simulink model "gm_Encoder_Zynq_vnl"  (R2018a)
settings: Solver=ode3  StartTime=0.0  StopTime=SimulationsDauer  RelTol=1e-3  EnableMultiTasking=on
undefined symbols (not defined in the file or in its folder): DiscIntNeverNeededParam, f_ISR, IncPerTurn, n_max, OverSamplingFactor, OverSamplingFactorInverse, Periode, Phase_Delay_A, Phase_Delay_B, PolePair, T_mech, TestDrehzahl_rpm
libraries: simulink x18, hdlsllib x2, dspsigops x2, dspswit3 x2, powerlib_meascontrol x2, hdlmdlgenlib x1, simulink_extras x1, powerlib x1
(part 3 of 3)

== system gm_Encoder_Zynq_vnl/IncreEncoder_V22/Check_Direction ==
  A : Inport  PortDimensions=1  SampleTime=2e-08
  B : Inport  Port=2  PortDimensions=1  SampleTime=2e-08
  Add : Sum  Inputs=+-  AccumDataTypeStr=fixdt(1, 4, 0)  OutDataTypeStr=fixdt(1, 4, 0)  SampleTime=2e-08
  Add1 : Sum  Inputs=+-  AccumDataTypeStr=fixdt(1, 4, 0)  OutDataTypeStr=fixdt(1, 4, 0)  SampleTime=2e-08
  Add2 : Sum  AccumDataTypeStr=fixdt(1, 4, 0)  OutDataTypeStr=fixdt(1, 4, 0)  SampleTime=2e-08
  Change : Sum  AccumDataTypeStr=fixdt(1, 4, 0)  OutDataTypeStr=fixdt(1, 4, 0)  SampleTime=2e-08
  Change1 : Delay  DelayLength=double(1)  InitialCondition=0  InputProcessing=Inherited  SampleTime=2e-08
  Save_Direction : Switch  Criteria=u2 ~= 0  Threshold=double(0)  OutDataTypeStr=fixdt(1, 4, 0)  SampleTime=2e-08
  T_count_switch : Switch  Threshold=double(1)  OutDataTypeStr=fixdt(1, 4, 0)  SampleTime=2e-08
  TrnLeft : Sum  Inputs=+-  AccumDataTypeStr=fixdt(1, 4, 0)  OutDataTypeStr=fixdt(1, 4, 0)  SampleTime=2e-08
  TrnRight : Sum  Inputs=+-  AccumDataTypeStr=fixdt(1, 4, 0)  OutDataTypeStr=fixdt(1, 4, 0)  SampleTime=2e-08
  TurnLeft : Constant  Value=fi(0,1,4,0,'hex','f')  OutDataTypeStr=fixdt(1, 4, 0)  SampleTime=-1
  TurnRight : Constant  Value=fi(0,1,4,0,'hex','1')  OutDataTypeStr=fixdt(1, 4, 0)  SampleTime=-1
  count_old : Delay  DelayLength=double(1)  InitialCondition=0  InputProcessing=Inherited  SampleTime=2e-08
  count_old1 : Delay  DelayLength=double(1)  InitialCondition=0  InputProcessing=Inherited  SampleTime=2e-08
  count_old2 : Delay  DelayLength=double(1)  InitialCondition=0  InputProcessing=Inherited  SampleTime=2e-08
  count_old_switch : Switch  Criteria=u2 ~= 0  Threshold=double(0)  OutDataTypeStr=boolean  SampleTime=2e-08
  count_old_switch1 : Switch  Criteria=u2 ~= 0  Threshold=double(0)  OutDataTypeStr=boolean  SampleTime=2e-08
  new_value : Delay  DelayLength=double(1)  InitialCondition=0  InputProcessing=Inherited  SampleTime=2e-08
  nothing : Constant  Value=fi(0,1,4,0,'hex','0')  OutDataTypeStr=fixdt(1, 4, 0)  SampleTime=-1
  nothing1 : Constant  Value=fi(0,1,4,0,'hex','0')  OutDataTypeStr=fixdt(1, 4, 0)  SampleTime=-1
  speed_old_switch : Switch  Threshold=double(1)  OutDataTypeStr=fixdt(1, 4, 0)  SampleTime=2e-08
  Dir : Outport
  wires:
  Save_Direction/1 -> count_old2/1
  count_old1/1 -> Add1/2, count_old_switch1/3
  count_old_switch1/1 -> count_old1/1
  count_old/1 -> Add/2, count_old_switch/3
  count_old_switch/1 -> count_old/1
  B/1 -> Add1/1, count_old_switch1/1, TrnRight/2
  A/1 -> Add/1, count_old_switch/1, TrnLeft/2
  speed_old_switch/1 -> Add2/2, Change/2
  nothing1/1 -> T_count_switch/3
  nothing/1 -> speed_old_switch/3
  new_value/1 -> Save_Direction/1
  count_old2/1 -> Save_Direction/3, Dir/1
  TurnRight/1 -> T_count_switch/1
  TurnLeft/1 -> speed_old_switch/1
  TrnRight/1 -> T_count_switch/2
  TrnLeft/1 -> speed_old_switch/2
  T_count_switch/1 -> Add2/1, Change/1
  Change1/1 -> Save_Direction/2
  Change/1 -> Change1/1
  Add2/1 -> new_value/1
  Add1/1 -> count_old_switch1/2, TrnLeft/1
  Add/1 -> count_old_switch/2, TrnRight/1

== system gm_Encoder_Zynq_vnl/IncreEncoder_V22/Counter ==
  note: 1 for one cycle if edge recognized
  note: Reset
  Enable_ctr : Inport  PortDimensions=1  SampleTime=2e-08
  I_line : Inport  Port=2  PortDimensions=1  SampleTime=2e-08
  Detec_edge : Sum  Inputs=+-  AccumDataTypeStr=int8  OutDataTypeStr=int8  SampleTime=2e-08
  Reset_flag : Sum  Inputs=+-  AccumDataTypeStr=uint8  OutDataTypeStr=uint8  SampleTime=2e-08
  reset_old : Delay  DelayLength=double(1)  InitialCondition=0  InputProcessing=Inherited  SampleTime=2e-08
  reset_old1 : Delay  DelayLength=double(1)  InitialCondition=0  InputProcessing=Inherited  SampleTime=2e-08
  reset_old_switch : Switch  Criteria=u2 ~= 0  Threshold=double(0)  OutDataTypeStr=boolean  SampleTime=2e-08
  reset_old_switch1 : Switch  Criteria=u2 ~= 0  Threshold=double(0)  OutDataTypeStr=boolean  SampleTime=2e-08
  Edge : Outport
  Reset : Outport  Port=2
  wires:
  reset_old/1 -> Reset_flag/2, reset_old_switch/3
  reset_old_switch/1 -> reset_old/1
  reset_old1/1 -> Detec_edge/2, reset_old_switch1/3
  reset_old_switch1/1 -> reset_old1/1
  I_line/1 -> Reset_flag/1, reset_old_switch/1
  Enable_ctr/1 -> Detec_edge/1, reset_old_switch1/1
  Detec_edge/1 -> reset_old_switch1/2, Edge/1
  Reset_flag/1 -> reset_old_switch/2, Reset/1

== system gm_Encoder_Zynq_vnl/IncreEncoder_V22/Counter_theta ==
  note: Count
  note: Check if count is to big
  note: Check if count is to small
  Edge : Inport  PortDimensions=1  SampleTime=2e-08
  Reset : Inport  Port=2  PortDimensions=1  SampleTime=2e-08
  IncsPerTurn : Inport  Port=3  PortDimensions=1  SampleTime=2e-08
  Dir : Inport  Port=4  PortDimensions=1  SampleTime=2e-08
  Add1 : Sum  AccumDataTypeStr=int16  OutDataTypeStr=int16  SampleTime=2e-08
  Constant1 : Constant  Value=fi(0,1,16,0,'hex','0000')  OutDataTypeStr=int16  SampleTime=-1
  Constant2 : Constant  Value=fi(0,1,16,0,'hex','0001')  OutDataTypeStr=int16  SampleTime=-1
  Constant3 : Constant  Value=fi(0,1,16,0,'hex','0000')  OutDataTypeStr=int16  SampleTime=-1
  Constant4 : Constant  Value=fi(0,1,16,0,'hex','000a')  OutDataTypeStr=int16  SampleTime=-1
  Constant5 : Constant  Value=fi(0,1,16,0,'hex','ffff')  OutDataTypeStr=int16  SampleTime=-1
  Relational Operator : RelationalOperator  Operator=>  OutDataTypeStr=boolean  SampleTime=2e-08  RndMeth=Nearest
  Relational Operator1 : RelationalOperator  Operator=<=  OutDataTypeStr=boolean  SampleTime=2e-08  RndMeth=Nearest
  Reset_when_overflow : Sum  AccumDataTypeStr=fixdt(1, 18, 0)  OutDataTypeStr=int16  SampleTime=2e-08
  Resett_switch1 : Switch  Criteria=u2 ~= 0  Threshold=double(0)  OutDataTypeStr=int16  SampleTime=2e-08
  Resett_switch2 : Switch  Criteria=u2 ~= 0  Threshold=double(0)  OutDataTypeStr=int16  SampleTime=2e-08
  Resett_switch3 : Switch  Criteria=u2 ~= 0  Threshold=double(0)  OutDataTypeStr=int16  SampleTime=2e-08
  delayMatch{,1..4} (5 alike) : Delay  DelayLength=double(1)  InitialCondition=0  InputProcessing=Inherited  SampleTime=2e-08
  only_use_for_neg_speed : Switch  Threshold=double(1)  OutDataTypeStr=int16  SampleTime=2e-08
  reset_old{2..6} (5 alike) : Delay  DelayLength=double(1)  InitialCondition=0  InputProcessing=Inherited  SampleTime=2e-08
  speed_old_switch1 : Switch  Criteria=u2 ~= 0  Threshold=double(0)  OutDataTypeStr=int16  SampleTime=2e-08
  speed_old_switch2 : Switch  Threshold=double(1)  OutDataTypeStr=int16  SampleTime=2e-08
  count : Outport
  wires:
  Resett_switch1/1 -> reset_old3/1
  Relational Operator/1 -> Resett_switch1/2
  Resett_switch3/1 -> reset_old2/1, Resett_switch1/3
  only_use_for_neg_speed/1 -> Resett_switch3/2
  Relational Operator1/1 -> only_use_for_neg_speed/3
  reset_old2/1 -> Relational Operator1/1
  Resett_switch2/1 -> Resett_switch3/3
  Add1/1 -> Resett_switch2/3
  Dir/1 -> reset_old6/1
  IncsPerTurn/1 -> Reset_when_overflow/2, delayMatch3/1
  Reset/1 -> delayMatch1/1
  Edge/1 -> speed_old_switch1/2
  reset_old3/1 -> Add1/2, Relational Operator/1, count/1
  reset_old5/1 -> delayMatch4/1
  reset_old6/1 -> speed_old_switch2/2, delayMatch2/1
  reset_old4/1 -> delayMatch/1
  speed_old_switch2/1 -> reset_old4/1
  speed_old_switch1/1 -> Add1/1
  delayMatch2/1 -> only_use_for_neg_speed/2
  delayMatch4/1 -> Relational Operator/2
  delayMatch/1 -> speed_old_switch1/1
  Reset_when_overflow/1 -> reset_old5/1
  Constant5/1 -> speed_old_switch2/3
  Constant4/1 -> Reset_when_overflow/1
  Constant3/1 -> speed_old_switch1/3
  Constant2/1 -> speed_old_switch2/1
  Constant1/1 -> Relational Operator1/2, Resett_switch1/1, Resett_switch2/1, only_use_for_neg_speed/1
  delayMatch3/1 -> Resett_switch3/1
  delayMatch1/1 -> Resett_switch2/2

== system gm_Encoder_Zynq_vnl/IncreEncoder_V22/Counter_theta_ele ==
  note: Count
  note: Check if count is to big
  note: Check if count is to small
  Edge : Inport  PortDimensions=1  SampleTime=2e-08
  Reset : Inport  Port=2  PortDimensions=1  SampleTime=2e-08
  IncsPerTurn : Inport  Port=3  PortDimensions=1  SampleTime=2e-08
  Dir : Inport  Port=4  PortDimensions=1  SampleTime=2e-08
  Add1 : Sum  AccumDataTypeStr=int16  OutDataTypeStr=int16  SampleTime=2e-08
  Constant1 : Constant  Value=fi(0,1,16,0,'hex','0000')  OutDataTypeStr=int16  SampleTime=-1
  Constant2 : Constant  Value=fi(0,1,16,0,'hex','0001')  OutDataTypeStr=int16  SampleTime=-1
  Constant3 : Constant  Value=fi(0,1,16,0,'hex','0000')  OutDataTypeStr=int16  SampleTime=-1
  Constant5 : Constant  Value=fi(0,1,16,0,'hex','ffff')  OutDataTypeStr=int16  SampleTime=-1
  Relational Operator : RelationalOperator  Operator=>  OutDataTypeStr=boolean  SampleTime=2e-08  RndMeth=Nearest
  Relational Operator1 : RelationalOperator  Operator=<=  OutDataTypeStr=boolean  SampleTime=2e-08  RndMeth=Nearest
  Resett_switch1 : Switch  Criteria=u2 ~= 0  Threshold=double(0)  OutDataTypeStr=int16  SampleTime=2e-08
  Resett_switch2 : Switch  Criteria=u2 ~= 0  Threshold=double(0)  OutDataTypeStr=int16  SampleTime=2e-08
  Resett_switch3 : Switch  Criteria=u2 ~= 0  Threshold=double(0)  OutDataTypeStr=int16  SampleTime=2e-08
  delayMatch{,1..3} (4 alike) : Delay  DelayLength=double(1)  InitialCondition=0  InputProcessing=Inherited  SampleTime=2e-08
  only_use_for_neg_speed : Switch  Threshold=double(1)  OutDataTypeStr=int16  SampleTime=2e-08
  reset_old{2..5} (4 alike) : Delay  DelayLength=double(1)  InitialCondition=0  InputProcessing=Inherited  SampleTime=2e-08
  speed_old_switch1 : Switch  Criteria=u2 ~= 0  Threshold=double(0)  OutDataTypeStr=int16  SampleTime=2e-08
  speed_old_switch2 : Switch  Threshold=double(1)  OutDataTypeStr=int16  SampleTime=2e-08
  count : Outport
  wires:
  Resett_switch1/1 -> reset_old3/1
  Relational Operator/1 -> Resett_switch1/2
  Resett_switch3/1 -> reset_old2/1, Resett_switch1/3
  only_use_for_neg_speed/1 -> Resett_switch3/2
  Relational Operator1/1 -> only_use_for_neg_speed/3
  reset_old2/1 -> Relational Operator1/1
  Resett_switch2/1 -> Resett_switch3/3
  Add1/1 -> Resett_switch2/3
  Dir/1 -> reset_old5/1
  IncsPerTurn/1 -> delayMatch3/1
  Reset/1 -> delayMatch1/1
  Edge/1 -> speed_old_switch1/2
  reset_old3/1 -> Add1/2, Relational Operator/1, count/1
  reset_old5/1 -> speed_old_switch2/2, delayMatch2/1
  reset_old4/1 -> delayMatch/1
  speed_old_switch2/1 -> reset_old4/1
  speed_old_switch1/1 -> Add1/1
  delayMatch2/1 -> only_use_for_neg_speed/2
  delayMatch/1 -> speed_old_switch1/1
  Constant5/1 -> speed_old_switch2/3
  Constant3/1 -> speed_old_switch1/3
  Constant2/1 -> speed_old_switch2/1
  Constant1/1 -> Relational Operator1/2, Resett_switch1/1, Resett_switch2/1, only_use_for_neg_speed/1
  delayMatch3/1 -> Relational Operator/2, Resett_switch3/1
  delayMatch1/1 -> Resett_switch2/2

== system gm_Encoder_Zynq_vnl/IncreEncoder_V22/HDL Reciprocal ==
  In1 : Inport
  Delay1 : Delay  DelayLength=1  InputProcessing=Inherited
  Delay2 : Delay  DelayLength=3  InputProcessing=Inherited
  HDL Reciprocal : Reciprocal  SampleTime=2e-08
  Out1 : Outport
  wires:
  Delay2/1 -> Out1/1
  HDL Reciprocal/1 -> Delay2/1
  Delay1/1 -> HDL Reciprocal/1
  In1/1 -> Delay1/1

== system gm_Encoder_Zynq_vnl/IncreEncoder_V22/Product_theta_el0_deserializer ==
  in0 : Inport  OutDataTypeStr=fixdt(0, 40, 24)  SampleTime=1e-08
  Product_theta_el0_deserializer : hdlsllib/HDL Operations/Deserializer1D  Ratio=2  IdleCycles=0  InitialCondition=double(0)  startIn=off  validIn=off  validOut=off  inputDataDimensions=1  inputSampleTime=1e-08  inputSignalType=real
      settings: SourceProductName=HDL Coder  SourceProductBaseCode=HD
  Product_theta_el0_deserializer_in_buff : SignalSpecification  OutDataTypeStr=fixdt(0, 40, 24)  Dimensions=1
  out0 : Outport  OutDataTypeStr=fixdt(0, 40, 24)  PortDimensions=[2]
  wires:
  Product_theta_el0_deserializer_in_buff/1 -> Product_theta_el0_deserializer/1
  in0/1 -> Product_theta_el0_deserializer_in_buff/1
  Product_theta_el0_deserializer/1 -> out0/1

== system gm_Encoder_Zynq_vnl/IncreEncoder_V22/Serializer_Subnetwork ==
  in0 : Inport  OutDataTypeStr=fixdt(0, 24, 24)  PortDimensions=[2]  SampleTime=2e-08
  in1 : Inport  Port=2  OutDataTypeStr=fixdt(0, 1, 0)  SampleTime=1e-08
  ratechange : dspsigops/Repeat  N=double(2)  RateOptions=Allow multirate processing  ic=0  mode=Unused parameter value
      settings: SourceProductName=DSP System Toolbox
  ratechange_splitcomp : Demux  Outputs=2
  splitcomp_multiport : MultiPortSwitch  DataPortOrder=Zero-based contiguous  Inputs=2  DiagnosticForDefault=None  zeroidx=on  OutDataTypeStr=fixdt(0, 24, 24)  SampleTime=1e-08
  out0 : Outport  OutDataTypeStr=fixdt(0, 24, 24)
  wires:
  in1/1 -> splitcomp_multiport/1
  in0/1 -> ratechange/1
  splitcomp_multiport/1 -> out0/1
  ratechange_splitcomp/2 -> splitcomp_multiport/3
  ratechange_splitcomp/1 -> splitcomp_multiport/2
  ratechange/1 -> ratechange_splitcomp/1

== system gm_Encoder_Zynq_vnl/IncreEncoder_V22/Serializer_Subnetwork1 ==
  in0 : Inport  OutDataTypeStr=uint16  PortDimensions=[2]  SampleTime=2e-08
  in1 : Inport  Port=2  OutDataTypeStr=fixdt(0, 1, 0)  SampleTime=1e-08
  ratechange : dspsigops/Repeat  N=double(2)  RateOptions=Allow multirate processing  ic=0  mode=Unused parameter value
      settings: SourceProductName=DSP System Toolbox
  ratechange_splitcomp : Demux  Outputs=2
  splitcomp_multiport : MultiPortSwitch  DataPortOrder=Zero-based contiguous  Inputs=2  DiagnosticForDefault=None  zeroidx=on  OutDataTypeStr=uint16  SampleTime=1e-08
  out0 : Outport  OutDataTypeStr=uint16
  wires:
  in1/1 -> splitcomp_multiport/1
  in0/1 -> ratechange/1
  splitcomp_multiport/1 -> out0/1
  ratechange_splitcomp/2 -> splitcomp_multiport/3
  ratechange_splitcomp/1 -> splitcomp_multiport/2
  ratechange/1 -> ratechange_splitcomp/1

== system gm_Encoder_Zynq_vnl/IncreEncoder_V22/omega_by_count_lines ==
  note: Set new counter value
  note: Check if count is to big in order to safe for value overflow
  note: Count
  Edge : Inport  PortDimensions=1  SampleTime=2e-08
  Reset1 : Inport  Port=2  PortDimensions=1  SampleTime=2e-08
  IncsPerTurn : Inport  Port=3  PortDimensions=1  SampleTime=2e-08
  Add1 : Sum  AccumDataTypeStr=int16  OutDataTypeStr=int16  SampleTime=2e-08
  Constant1 : Constant  Value=fi(0,1,16,0,'hex','0000')  OutDataTypeStr=int16  SampleTime=-1
  Constant2 : Constant  Value=fi(0,1,16,0,'hex','0001')  OutDataTypeStr=int16  SampleTime=-1
  Constant3 : Constant  Value=fi(0,1,16,0,'hex','0000')  OutDataTypeStr=int16  SampleTime=-1
  Constant4 : Constant  Value=fi(0,1,16,0,'hex','000a')  OutDataTypeStr=int16  SampleTime=-1
  Relational Operator : RelationalOperator  Operator=>  OutDataTypeStr=boolean  SampleTime=2e-08  RndMeth=Nearest
  Reset_when_overflow : Sum  AccumDataTypeStr=fixdt(1, 18, 0)  OutDataTypeStr=int16  SampleTime=2e-08
  Resett_switch1 : Switch  Criteria=u2 ~= 0  Threshold=double(0)  OutDataTypeStr=int16  SampleTime=2e-08
  Resett_switch2 : Switch  Criteria=u2 ~= 0  Threshold=double(0)  OutDataTypeStr=int16  SampleTime=2e-08
  delayMatch{,1..3} (4 alike) : Delay  DelayLength=double(1)  InitialCondition=0  InputProcessing=Inherited  SampleTime=2e-08
  reset_old{1,3..5} (4 alike) : Delay  DelayLength=double(1)  InitialCondition=0  InputProcessing=Inherited  SampleTime=2e-08
  reset_old_switch1 : Switch  Criteria=u2 ~= 0  Threshold=double(0)  OutDataTypeStr=int16  SampleTime=2e-08
  speed_old_switch1 : Switch  Criteria=u2 ~= 0  Threshold=double(0)  OutDataTypeStr=int16  SampleTime=2e-08
  count : Outport
  wires:
  reset_old1/1 -> reset_old_switch1/3
  Resett_switch1/1 -> reset_old3/1
  Relational Operator/1 -> Resett_switch1/2
  Resett_switch2/1 -> Resett_switch1/3
  Add1/1 -> Resett_switch2/3
  IncsPerTurn/1 -> Reset_when_overflow/2
  Reset1/1 -> delayMatch1/1, delayMatch3/1
  Edge/1 -> speed_old_switch1/2
  reset_old_switch1/1 -> reset_old1/1, count/1
  reset_old3/1 -> reset_old_switch1/1, Add1/2, Relational Operator/1
  reset_old5/1 -> delayMatch2/1
  delayMatch3/1 -> reset_old_switch1/2
  reset_old4/1 -> delayMatch/1
  speed_old_switch1/1 -> Add1/1
  delayMatch2/1 -> Relational Operator/2
  delayMatch/1 -> speed_old_switch1/1
  Reset_when_overflow/1 -> reset_old5/1
  Constant4/1 -> Reset_when_overflow/1
  Constant3/1 -> speed_old_switch1/3
  Constant2/1 -> reset_old4/1
  Constant1/1 -> Resett_switch1/1, Resett_switch2/1
  delayMatch1/1 -> Resett_switch2/2

== system gm_Encoder_Zynq_vnl/IncreEncoder_V22/omega_by_measure_time ==
  note: Count up in order to measure the time between to positive edges of the A-Line of the encoder
  note: Reset time measurement
  note: Detect each positive edge of the A-Line of the encoder
  note: 1 for one cycle if edge recognized
  note: Use new Speed after every positive A-Line Edge
  Edge : Inport  PortDimensions=1  SampleTime=2e-08
  T : Inport  Port=2  PortDimensions=1  SampleTime=2e-08
  Add1 : Sum  AccumDataTypeStr=fixdt(0, 32, 26)  OutDataTypeStr=fixdt(0, 32, 26)  SampleTime=2e-08
  Add1_out1 : hdlmdlgenlib/Buffer
      settings: SourceProductName=HDL Coder  SourceProductBaseCode=HD
  Constant : Constant  Value=fi(0,0,32,26,'hex','00000000')  OutDataTypeStr=fixdt(0, 32, 26)  SampleTime=-1
  Constant1 : Constant  Value=fi(0,0,32,26,'hex','00000000')  OutDataTypeStr=fixdt(0, 32, 26)  SampleTime=-1
  Constant2 : Constant  Value=fi(0,0,32,26,'hex','00000000')  OutDataTypeStr=fixdt(0, 32, 26)  SampleTime=-1
  Constant3 : Constant  Value=fi(0,1,8,0,'hex','00')  OutDataTypeStr=int8  SampleTime=-1
  Detec_edge : Sum  Inputs=+-  AccumDataTypeStr=int8  OutDataTypeStr=int8  SampleTime=2e-08
  ProtectOverflow_T_count : Switch  Threshold=double(50)  OutDataTypeStr=fixdt(0, 32, 26)  SampleTime=2e-08
  ProtectOverflow_rps : Switch  Threshold=double(50)  OutDataTypeStr=fixdt(0, 32, 26)  SampleTime=2e-08
  ProtectToUseOmegaIfThetaJump1 : RelationalOperator  Operator=>  OutDataTypeStr=boolean  SampleTime=2e-08  RndMeth=Nearest
  Scope : Scope  NumInputPorts=3
  T_count : Delay  DelayLength=double(1)  InitialCondition=0  InputProcessing=Inherited  SampleTime=2e-08
  T_count_switch : Switch  Criteria=u2 > Threshold  Threshold=double(0)  OutDataTypeStr=fixdt(0, 32, 26)  SampleTime=2e-08
  count_old1 : Delay  DelayLength=double(1)  InitialCondition=0  InputProcessing=Inherited  SampleTime=2e-08
  delayMatch : Delay  DelayLength=double(1)  InitialCondition=0  InputProcessing=Inherited  SampleTime=2e-08
  reset_old1 : Delay  DelayLength=double(1)  InitialCondition=0  InputProcessing=Inherited  SampleTime=2e-08
  reset_old_switch1 : Switch  Criteria=u2 ~= 0  Threshold=double(0)  OutDataTypeStr=boolean  SampleTime=2e-08
  speed_old : Delay  DelayLength=double(1)  InitialCondition=0  InputProcessing=Inherited  SampleTime=2e-08
  speed_old_switch : Switch  Criteria=u2 ~= 0  Threshold=double(0)  OutDataTypeStr=fixdt(0, 32, 26)  RndMeth=Zero  SampleTime=2e-08
  rps : Outport
  NewMeasurement : Outport  Port=2
  wires:
  speed_old/1 -> speed_old_switch/3
  T_count/1 -> Add1/2
  ProtectOverflow_T_count/1 -> T_count/1
  reset_old1/1 -> Detec_edge/2, reset_old_switch1/3
  reset_old_switch1/1 -> reset_old1/1
  T/1 -> delayMatch/1
  Edge/1 -> Detec_edge/1, reset_old_switch1/1
  speed_old_switch/1 -> speed_old/1, ProtectOverflow_rps/3
  T_count_switch/1 -> ProtectOverflow_T_count/2, ProtectOverflow_T_count/3, ProtectOverflow_rps/2
  Add1/1 -> T_count_switch/3, Add1_out1/1
  Detec_edge/1 -> reset_old_switch1/2, count_old1/1
  count_old1/1 -> ProtectToUseOmegaIfThetaJump1/1
  ProtectToUseOmegaIfThetaJump1/1 -> speed_old_switch/2, T_count_switch/2, NewMeasurement/1, Scope/1
  ProtectOverflow_rps/1 -> rps/1, Scope/3
  Constant3/1 -> ProtectToUseOmegaIfThetaJump1/2
  Constant2/1 -> ProtectOverflow_rps/1
  Constant1/1 -> ProtectOverflow_T_count/1
  Constant/1 -> T_count_switch/1
  Add1_out1/1 -> speed_old_switch/1, Scope/2
  delayMatch/1 -> Add1/1

== system gm_Encoder_Zynq_vnl/IncreEncoder_V22_vnl/Average ==
  note: Maximum of the OverSampling is 6
  "OmegaIn " : Inport
  NewMeasurement : Inport  Port=2
  SamplingFactorInv : Inport  Port=3
  SamplingFactor : Inport  Port=4
  Add : Sum  Inputs=++++++  OutDataTypeStr=Inherit: Same as first input
  Ask1 : Switch  Threshold=fi(2,0,4,0)  OutDataTypeStr=fixdt(1,24,11)
  Ask2 : Switch  Threshold=fi(3,0,4,0)  OutDataTypeStr=fixdt(1,24,11)
  Ask3 : Switch  Threshold=fi(4,0,4,0)  OutDataTypeStr=fixdt(1,24,11)
  Ask4 : Switch  Threshold=fi(5,0,4,0)  OutDataTypeStr=fixdt(1,24,11)
  Ask5 : Switch  Threshold=fi(6,0,4,0)  OutDataTypeStr=fixdt(1,24,11)
  Constant1 : Constant  Value=0  OutDataTypeStr=fixdt(1,24,11)  SampleTime=-1
  NewSpeed{,1..4} (5 alike) : Switch  Criteria=u2 ~= 0  Threshold=0.5  OutDataTypeStr=fixdt(1,24,11)
  Product : Product  OutDataTypeStr=Inherit: Same as first input
  hold{,1..4} (5 alike) : Delay  DelayLength=1
  OmegaOut : Outport
  wires:
  SamplingFactor/1 -> Ask5/2, Ask4/2, Ask3/2, Ask2/2, Ask1/2
  Ask5/1 -> Add/6
  Ask4/1 -> Add/5
  Ask3/1 -> Add/4
  Ask2/1 -> Add/3
  Ask1/1 -> Add/2
  Constant1/1 -> Ask1/3, Ask2/3, Ask3/3, Ask4/3, Ask5/3
  hold4/1 -> NewSpeed4/3
  NewSpeed4/1 -> Ask5/1, hold4/1
  hold3/1 -> NewSpeed3/3, NewSpeed4/1
  NewSpeed3/1 -> Ask4/1, hold3/1
  NewMeasurement/1 -> NewSpeed/2, NewSpeed1/2, NewSpeed2/2, NewSpeed3/2, NewSpeed4/2
  NewSpeed2/1 -> Ask3/1, hold2/1
  hold2/1 -> NewSpeed2/3, NewSpeed3/1
  hold1/1 -> NewSpeed1/3, NewSpeed2/1
  NewSpeed1/1 -> Ask2/1, hold1/1
  NewSpeed/1 -> Ask1/1, hold/1
  hold/1 -> NewSpeed/3, NewSpeed1/1
  Add/1 -> Product/1
  SamplingFactorInv/1 -> Product/2
  "OmegaIn "/1 -> NewSpeed/1, Add/1
  Product/1 -> OmegaOut/1

== system gm_Encoder_Zynq_vnl/IncreEncoder_V22_vnl/Check_Direction ==
  A : Inport
  B : Inport  Port=2
  Add : Sum  Inputs=+-  AccumDataTypeStr=fixdt(1,4,0)  OutDataTypeStr=fixdt(1,4,0)
  Add1 : Sum  Inputs=+-  AccumDataTypeStr=fixdt(1,4,0)  OutDataTypeStr=fixdt(1,4,0)
  Add2 : Sum  AccumDataTypeStr=fixdt(1,4,0)  OutDataTypeStr=fixdt(1,4,0)
  Change : Sum  AccumDataTypeStr=fixdt(1,4,0)  OutDataTypeStr=fixdt(1,4,0)
  Change1 : Delay  DelayLength=1
  Save_Direction : Switch  Criteria=u2 ~= 0  Threshold=0.1  OutDataTypeStr=Inherit: Inherit via back propagation
  T_count_switch : Switch  Threshold=1  OutDataTypeStr=Inherit: Inherit via back propagation
  TrnLeft : Sum  Inputs=+-  AccumDataTypeStr=fixdt(1,4,0)  OutDataTypeStr=fixdt(1,4,0)
  TrnRight : Sum  Inputs=+-  AccumDataTypeStr=fixdt(1,4,0)  OutDataTypeStr=fixdt(1,4,0)
  TurnLeft : Constant  Value=-1  OutDataTypeStr=fixdt(1,4,0)  SampleTime=-1
  TurnRight : Constant  OutDataTypeStr=fixdt(1,4,0)  SampleTime=-1
  count_old : Delay  DelayLength=1
  count_old1 : Delay  DelayLength=1
  count_old2 : Delay  DelayLength=1
  count_old_switch : Switch  Criteria=u2 ~= 0  OutDataTypeStr=Inherit: Inherit via back propagation
  count_old_switch1 : Switch  Criteria=u2 ~= 0  OutDataTypeStr=Inherit: Inherit via back propagation
  new_value : Delay  DelayLength=1
  nothing : Constant  Value=0  OutDataTypeStr=fixdt(1,4,0)  SampleTime=-1
  nothing1 : Constant  Value=0  OutDataTypeStr=fixdt(1,4,0)  SampleTime=-1
  speed_old_switch : Switch  Threshold=1  OutDataTypeStr=Inherit: Inherit via back propagation
  Dir : Outport
  wires:
  count_old2/1 -> Dir/1, Save_Direction/3
  Change1/1 -> Save_Direction/2
  Change/1 -> Change1/1
  Add2/1 -> new_value/1
  speed_old_switch/1 -> Add2/2, Change/2
  nothing1/1 -> T_count_switch/3
  nothing/1 -> speed_old_switch/3
  TurnLeft/1 -> speed_old_switch/1
  TrnLeft/1 -> speed_old_switch/2
  new_value/1 -> Save_Direction/1
  TrnRight/1 -> T_count_switch/2
  Add1/1 -> count_old_switch1/2, TrnLeft/1
  count_old1/1 -> Add1/2, count_old_switch1/3
  count_old_switch1/1 -> count_old1/1
  B/1 -> count_old_switch1/1, Add1/1, TrnRight/2
  Save_Direction/1 -> count_old2/1
  T_count_switch/1 -> Add2/1, Change/1
  Add/1 -> count_old_switch/2, TrnRight/1
  TurnRight/1 -> T_count_switch/1
  count_old/1 -> Add/2, count_old_switch/3
  count_old_switch/1 -> count_old/1
  A/1 -> count_old_switch/1, Add/1, TrnLeft/2

== system gm_Encoder_Zynq_vnl/IncreEncoder_V22_vnl/Counter ==
  note: Reset
  note: 1 for one cycle if edge recognized
  Enable_ctr : Inport
  I_line : Inport  Port=2
  Detec_edge : Sum  Inputs=+-  AccumDataTypeStr=int8  OutDataTypeStr=int8
  Reset_flag : Sum  Inputs=+-  AccumDataTypeStr=uint8  OutDataTypeStr=uint8
  reset_old : Delay  DelayLength=1
  reset_old1 : Delay  DelayLength=1
  reset_old_switch : Switch  Criteria=u2 ~= 0
  reset_old_switch1 : Switch  Criteria=u2 ~= 0
  Edge : Outport
  Reset : Outport  Port=2
  wires:
  Detec_edge/1 -> Edge/1, reset_old_switch1/2  "1 for one cycle if edge recognized"
  reset_old1/1 -> Detec_edge/2, reset_old_switch1/3
  reset_old_switch1/1 -> reset_old1/1
  Enable_ctr/1 -> reset_old_switch1/1, Detec_edge/1
  Reset_flag/1 -> reset_old_switch/2, Reset/1
  reset_old/1 -> Reset_flag/2, reset_old_switch/3
  reset_old_switch/1 -> reset_old/1
  I_line/1 -> reset_old_switch/1, Reset_flag/1

== system gm_Encoder_Zynq_vnl/IncreEncoder_V22_vnl/Counter_theta ==
  note: Check if count is to small
  note: Check if count is to big
  note: Count
  Edge : Inport
  Reset : Inport  Port=2
  IncsPerTurn : Inport  Port=3
  Dir : Inport  Port=4
  Add1 : Sum  AccumDataTypeStr=int16  OutDataTypeStr=int16
  Constant1 : Constant  Value=0  OutDataTypeStr=int16  SampleTime=-1
  Constant2 : Constant  OutDataTypeStr=int16  SampleTime=-1
  Constant3 : Constant  Value=0  OutDataTypeStr=int16  SampleTime=-1
  Constant4 : Constant  Value=10  OutDataTypeStr=int16  SampleTime=-1
  Constant5 : Constant  Value=-1  OutDataTypeStr=int16  SampleTime=-1
  Relational Operator : RelationalOperator  Operator=>  OutDataTypeStr=boolean  RndMeth=Nearest
  Relational Operator1 : RelationalOperator  Operator=<=  OutDataTypeStr=boolean  RndMeth=Nearest
  Reset_when_overflow : Sum  OutDataTypeStr=int16
  Resett_switch1 : Switch  Criteria=u2 ~= 0  OutDataTypeStr=int16
  Resett_switch2 : Switch  Criteria=u2 ~= 0  OutDataTypeStr=int16
  Resett_switch3 : Switch  Criteria=u2 ~= 0  OutDataTypeStr=int16
  only_use_for_neg_speed : Switch  Threshold=1
  reset_old{2..6} (5 alike) : Delay  DelayLength=1
  speed_old_switch1 : Switch  Criteria=u2 ~= 0
  speed_old_switch2 : Switch  Threshold=1
  count : Outport
  wires:
  reset_old6/1 -> speed_old_switch2/2, only_use_for_neg_speed/2
  reset_old5/1 -> Relational Operator/2
  reset_old4/1 -> speed_old_switch1/1
  only_use_for_neg_speed/1 -> Resett_switch3/2
  Relational Operator1/1 -> only_use_for_neg_speed/3
  reset_old2/1 -> Relational Operator1/1
  Resett_switch2/1 -> Resett_switch3/3
  Resett_switch3/1 -> Resett_switch1/3, reset_old2/1
  Constant1/1 -> Relational Operator1/2, only_use_for_neg_speed/1, Resett_switch1/1, Resett_switch2/1
  Relational Operator/1 -> Resett_switch1/2
  Resett_switch1/1 -> reset_old3/1
  reset_old3/1 -> Relational Operator/1, count/1, Add1/2
  speed_old_switch2/1 -> reset_old4/1
  Constant5/1 -> speed_old_switch2/3
  Dir/1 -> reset_old6/1
  IncsPerTurn/1 -> Reset_when_overflow/2, Resett_switch3/1
  Reset_when_overflow/1 -> reset_old5/1
  Constant4/1 -> Reset_when_overflow/1
  Constant2/1 -> speed_old_switch2/1
  Constant3/1 -> speed_old_switch1/3
  speed_old_switch1/1 -> Add1/1
  Add1/1 -> Resett_switch2/3
  Edge/1 -> speed_old_switch1/2  "1 for one cycle if edge recognized"
  Reset/1 -> Resett_switch2/2

== system gm_Encoder_Zynq_vnl/IncreEncoder_V22_vnl/Counter_theta_ele ==
  note: Check if count is to small
  note: Check if count is to big
  note: Count
  Edge : Inport
  Reset : Inport  Port=2
  IncsPerTurn : Inport  Port=3
  Dir : Inport  Port=4
  Add1 : Sum  AccumDataTypeStr=int16  OutDataTypeStr=int16
  Constant1 : Constant  Value=0  OutDataTypeStr=int16  SampleTime=-1
  Constant2 : Constant  OutDataTypeStr=int16  SampleTime=-1
  Constant3 : Constant  Value=0  OutDataTypeStr=int16  SampleTime=-1
  Constant5 : Constant  Value=-1  OutDataTypeStr=int16  SampleTime=-1
  Relational Operator : RelationalOperator  Operator=>  OutDataTypeStr=boolean  RndMeth=Nearest
  Relational Operator1 : RelationalOperator  Operator=<=  OutDataTypeStr=boolean  RndMeth=Nearest
  Resett_switch1 : Switch  Criteria=u2 ~= 0  OutDataTypeStr=int16
  Resett_switch2 : Switch  Criteria=u2 ~= 0  OutDataTypeStr=int16
  Resett_switch3 : Switch  Criteria=u2 ~= 0  OutDataTypeStr=int16
  only_use_for_neg_speed : Switch  Threshold=1
  reset_old{2..5} (4 alike) : Delay  DelayLength=1
  speed_old_switch1 : Switch  Criteria=u2 ~= 0
  speed_old_switch2 : Switch  Threshold=1
  count : Outport
  wires:
  reset_old5/1 -> only_use_for_neg_speed/2, speed_old_switch2/2
  reset_old4/1 -> speed_old_switch1/1
  only_use_for_neg_speed/1 -> Resett_switch3/2
  Relational Operator1/1 -> only_use_for_neg_speed/3
  reset_old2/1 -> Relational Operator1/1
  Resett_switch2/1 -> Resett_switch3/3
  Resett_switch3/1 -> Resett_switch1/3, reset_old2/1
  Constant1/1 -> Resett_switch1/1, Relational Operator1/2, only_use_for_neg_speed/1, Resett_switch2/1
  Relational Operator/1 -> Resett_switch1/2
  Resett_switch1/1 -> reset_old3/1
  reset_old3/1 -> Relational Operator/1, count/1, Add1/2
  speed_old_switch2/1 -> reset_old4/1
  Constant5/1 -> speed_old_switch2/3
  Dir/1 -> reset_old5/1
  IncsPerTurn/1 -> Resett_switch3/1, Relational Operator/2
  Constant2/1 -> speed_old_switch2/1
  Constant3/1 -> speed_old_switch1/3
  speed_old_switch1/1 -> Add1/1
  Add1/1 -> Resett_switch2/3
  Edge/1 -> speed_old_switch1/2  "1 for one cycle if edge recognized"
  Reset/1 -> Resett_switch2/2

== system gm_Encoder_Zynq_vnl/IncreEncoder_V22_vnl/omega_by_count_lines ==
  note: Count
  note: Check if count is to big in order to safe for value overflow
  note: Set new counter value
  Edge : Inport
  Reset1 : Inport  Port=2
  IncsPerTurn : Inport  Port=3
  Add1 : Sum  AccumDataTypeStr=int16  OutDataTypeStr=int16
  Constant1 : Constant  Value=0  OutDataTypeStr=int16  SampleTime=-1
  Constant2 : Constant  OutDataTypeStr=int16  SampleTime=-1
  Constant3 : Constant  Value=0  OutDataTypeStr=int16  SampleTime=-1
  Constant4 : Constant  Value=10  OutDataTypeStr=int16  SampleTime=-1
  Relational Operator : RelationalOperator  Operator=>  OutDataTypeStr=boolean  RndMeth=Nearest
  Reset_when_overflow : Sum  OutDataTypeStr=int16
  Resett_switch1 : Switch  Criteria=u2 ~= 0  OutDataTypeStr=int16
  Resett_switch2 : Switch  Criteria=u2 ~= 0  OutDataTypeStr=int16
  reset_old{1,3..5} (4 alike) : Delay  DelayLength=1
  reset_old_switch1 : Switch  Criteria=u2 ~= 0
  speed_old_switch1 : Switch  Criteria=u2 ~= 0
  count : Outport
  wires:
  reset_old_switch1/1 -> count/1, reset_old1/1
  Reset1/1 -> Resett_switch2/2, reset_old_switch1/2  "Use new value"
  reset_old1/1 -> reset_old_switch1/3
  reset_old3/1 -> Relational Operator/1, Add1/2, reset_old_switch1/1
  Resett_switch1/1 -> reset_old3/1
  Constant4/1 -> Reset_when_overflow/1
  Constant2/1 -> reset_old4/1
  Add1/1 -> Resett_switch2/3
  IncsPerTurn/1 -> Reset_when_overflow/2
  Constant3/1 -> speed_old_switch1/3
  Constant1/1 -> Resett_switch1/1, Resett_switch2/1
  Edge/1 -> speed_old_switch1/2  "1 for one cycle if edge recognized"
  reset_old4/1 -> speed_old_switch1/1
  Resett_switch2/1 -> Resett_switch1/3
  reset_old5/1 -> Relational Operator/2
  speed_old_switch1/1 -> Add1/1
  Relational Operator/1 -> Resett_switch1/2
  Reset_when_overflow/1 -> reset_old5/1

== system gm_Encoder_Zynq_vnl/IncreEncoder_V22_vnl/omega_by_measure_time ==
  note: Use new Speed after every positive A-Line Edge
  note: 1 for one cycle if edge recognized
  note: Detect each positive edge of the A-Line of the encoder
  note: Reset time measurement
  note: Count up in order to measure the time between to positive edges of the A-Line of the encoder
  Edge : Inport
  T : Inport  Port=2
  Add1 : Sum  OutDataTypeStr=Inherit: Same as first input
  Constant : Constant  Value=0  OutDataTypeStr=fixdt(0,32,26)  SampleTime=-1
  Constant1 : Constant  Value=0  OutDataTypeStr=fixdt(0,32,26)  SampleTime=-1
  Constant2 : Constant  Value=0  OutDataTypeStr=fixdt(0,32,26)  SampleTime=-1
  Constant3 : Constant  Value=0  OutDataTypeStr=int8  SampleTime=-1
  Detec_edge : Sum  Inputs=+-  AccumDataTypeStr=int8  OutDataTypeStr=int8
  ProtectOverflow_T_count : Switch  Threshold=50
  ProtectOverflow_rps : Switch  Threshold=50  OutDataTypeStr=fixdt(0,32,26)
  ProtectToUseOmegaIfThetaJump1 : RelationalOperator  Operator=>  OutDataTypeStr=boolean  RndMeth=Nearest
  Scope : Scope  NumInputPorts=3
  T_count : Delay  DelayLength=1
  T_count_switch : Switch  Criteria=u2 > Threshold
  count_old1 : Delay  DelayLength=1
  reset_old1 : Delay  DelayLength=1
  reset_old_switch1 : Switch  Criteria=u2 ~= 0
  speed_old : Delay  DelayLength=1
  speed_old_switch : Switch  Criteria=u2 ~= 0  OutDataTypeStr=fixdt(0,32,26)  RndMeth=Zero
  rps : Outport
  NewMeasurement : Outport  Port=2
  wires:
  Detec_edge/1 -> reset_old_switch1/2, count_old1/1  "1 for one cycle if edge recognized"
  reset_old1/1 -> Detec_edge/2, reset_old_switch1/3
  reset_old_switch1/1 -> reset_old1/1
  Edge/1 -> Detec_edge/1, reset_old_switch1/1
  ProtectToUseOmegaIfThetaJump1/1 -> T_count_switch/2, speed_old_switch/2, NewMeasurement/1, Scope/1
  Constant3/1 -> ProtectToUseOmegaIfThetaJump1/2
  count_old1/1 -> ProtectToUseOmegaIfThetaJump1/1
  T_count_switch/1 -> ProtectOverflow_T_count/2, ProtectOverflow_T_count/3, ProtectOverflow_rps/2
  Add1/1 -> T_count_switch/3, speed_old_switch/1, Scope/2
  T_count/1 -> Add1/2
  ProtectOverflow_T_count/1 -> T_count/1
  T/1 -> Add1/1
  speed_old/1 -> speed_old_switch/3
  speed_old_switch/1 -> speed_old/1, ProtectOverflow_rps/3
  Constant2/1 -> ProtectOverflow_rps/1
  ProtectOverflow_rps/1 -> rps/1, Scope/3
  Constant1/1 -> ProtectOverflow_T_count/1
  Constant/1 -> T_count_switch/1

== system gm_Encoder_Zynq_vnl/IncrementalEncoder_Floating/CutTheta_0_2PI ==
  In1 : Inport
  Add7 : Sum  Inputs=+-  OutDataTypeStr=double
  Gain : Gain  Gain=1/(2*pi)
  Gain11 : Gain  Gain=2*pi
  Rounding Function : Rounding
  Out1 : Outport
  wires:
  Gain/1 -> Rounding Function/1
  Rounding Function/1 -> Gain11/1
  Gain11/1 -> Add7/2
  In1/1 -> Gain/1, Add7/1
  Add7/1 -> Out1/1

== system gm_Encoder_Zynq_vnl/IncrementalEncoder_Floating/n_aus_theta_v4 ==
  theta : Inport
  Abs : Abs
  Add : Sum  Inputs=-+
  Add1 : Sum  Inputs=+-
  Gain : Gain  Gain=2*pi
  Gain1 : Gain  Gain=1/T_mech
  Gain2 : Gain  Gain=60/(2*pi)
  Geschwindigkeitsfilter1 : Subsystem
  Rate Limiter2 1/T : RateLimiter  RisingSlewLimit=1/T_mech*10  FallingSlewLimit=-1/T_mech*10  SampleTimeMode=inherited
  Saturation : Saturate  UpperLimit=n_max  LowerLimit=-n_max
  Scope1 : Scope  NumInputPorts=5
  Scope2 : Scope  NumInputPorts=5
  Sign : Signum
  Switch : Switch  Threshold=3
  Unit Delay : UnitDelay  SampleTime=-1
  n : Outport
  wires:
  Switch/1 -> Scope1/3, Gain1/1
  Add/1 -> Scope2/1, Switch/1
  Gain/1 -> Add/1
  Sign/1 -> Gain/1
  Add1/1 -> Scope2/3, Add/2, Abs/1, Scope2/2, Switch/3, Sign/1
  Abs/1 -> Scope1/4, Switch/2
  Gain1/1 -> Scope1/2, Gain2/1
  theta/1 -> Scope2/5, Add1/1, Unit Delay/1
  Unit Delay/1 -> Scope2/4, Add1/2
  Gain2/1 -> Saturation/1
  Geschwindigkeitsfilter1/1(Out1) -> Scope1/5, Rate Limiter2 1/T/1
  Rate Limiter2 1/T/1 -> n/1
  Saturation/1 -> Scope1/1, Geschwindigkeitsfilter1/1(In1)

== system gm_Encoder_Zynq_vnl/IncrementalEncoder_Floating/n_aus_theta_v4/Geschwindigkeitsfilter1 ==
  In1 : Inport
  Add1 : Sum  Inputs=+-
  Discrete-Time Integrator2 : DiscreteIntegrator  SampleTime=-1  ICPrevOutput=DiscIntNeverNeededParam  ICPrevScaledInput=DiscIntNeverNeededParam
  Gain2 2500 10000 : Gain  Gain=10000
  Scope1 : Scope  NumInputPorts=5
  Out1 : Outport  InitialOutput=[0]
  wires:
  Add1/1 -> Scope1/4, Gain2 2500 10000/1
  Gain2 2500 10000/1 -> Scope1/3, Discrete-Time Integrator2/1
  Discrete-Time Integrator2/1 -> Scope1/2, Out1/1, Add1/2
  In1/1 -> Scope1/5, Add1/1
